simulink model "motorPI"  (R2026a)
settings: Solver=VariableStepAuto  MaxStep=1e-4
values from neighbouring files (symbols this model uses):
  den = [4.84323072847e-08 4.8661333765e-05 8.000321026e-05]    [piDesign.mat]    (also in transferFunction.m = conv([L R], [J D]) + [0 0 K^2])
  Kp = 0.2    [piDesign.m]    (also in piDesign.mat)
  num = 0.00868283239801    [piDesign.mat]    (also in transferFunction.m = K)
  T = 0.01    [piDesign.mat]    (also in transferFunction.m)
  tau_i = 1.0    (= 1)    [piDesign.m]    (also in piDesign.mat)
  Vmax = 8    [piDesign.m]    (also in piDesign.mat)
settings Model: Creator=bidaze  LastModifiedBy=bidaze

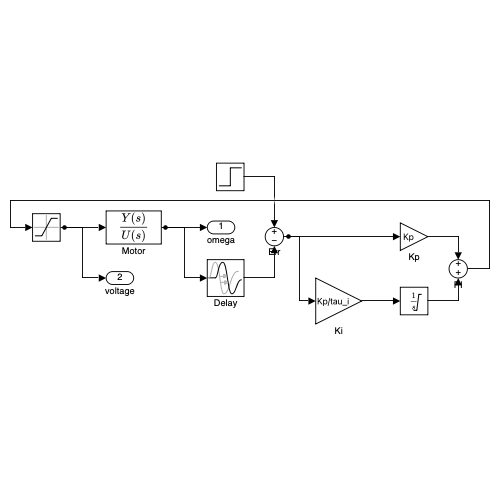
[thumbnail: Simulink's stored preview of the top-level diagram]
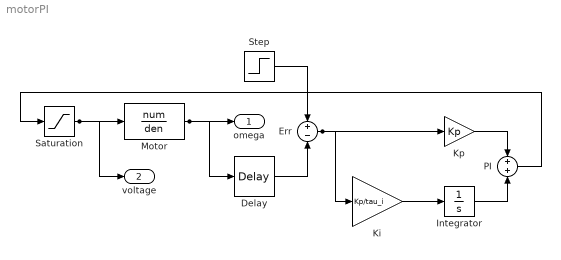
== system motorPI ==
  Delay : TransportDelay  DelayTime=T
  Err : Sum  Inputs=+-
  Integrator : Integrator  LimitOutput=on  UpperSaturationLimit=Vmax  LowerSaturationLimit=-Vmax
  Ki : Gain  Gain=Kp/tau_i
  Kp : Gain  Gain=Kp
  Motor : TransferFcn  Numerator=num  Denominator=den
  PI : Sum
  Saturation : Saturate  UpperLimit=Vmax  LowerLimit=-Vmax
  Step : Step  Time=0.1  FinalValue=wRef  SampleTime=0
  omega : Outport
  voltage : Outport  Port=2
  wires:
  Kp/1 -> PI/1
  Ki/1 -> Integrator/1
  Integrator/1 -> PI/2
  Delay/1 -> Err/2
  Err/1 -> Ki/1, Kp/1
  PI/1 -> Saturation/1
  Step/1 -> Err/1
  Motor/1 -> omega/1, Delay/1
  Saturation/1 -> voltage/1, Motor/1
